simulink model "dnm_10_0"  (R2015a)
settings: Solver=ode3  StartTime=0.0  StopTime=100  FixedStep=0.001  RelTol=1e-3
libraries: slident x1, simulink x1
settings Model: Creator=Administrator  LastModifiedBy=Administrator
settings DataIOCC: LimitDataPoints=off

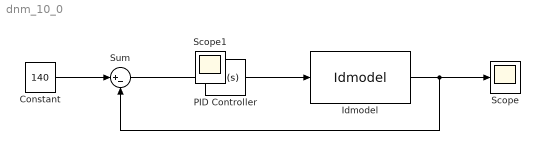
== system dnm_10_0 ==
  Constant : Constant  Value=140
  Idmodel : slident/Models/Idmodel  sys=P1Dc_10_0  IC=0  noi=off  seed=[]
  PID Controller : simulink/Continuous/PID Controller  Controller=PID  TimeDomain=Continuous-time  SampleTime=-1  IntegratorMethod=Forward Euler  FilterMethod=Forward Euler  Form=Parallel  UseFilter=on  ControllerParametersSource=internal  P=0.093556670716069  I=0.00376519243488328  D=0  N=100  InitialConditionSource=internal  InitialConditionForIntegrator=0  InitialConditionForFilter=0  ExternalReset=none  LimitOutput=off  UpperSaturationLimit=inf  LowerSaturationLimit=-inf  LinearizeAsGain=on  AntiWindupMode=none  Kb=1  TrackingMode=off  Kt=1  PParamMin=[]  PParamMax=[]  IParamMin=[]  IParamMax=[]  DParamMin=[]  DParamMax=[]  NParamMin=[]  NParamMax=[]  KbParamMin=[]  KbParamMax=[]  KtParamMin=[]  KtParamMax=[]  POutMin=[]  POutMax=[]  IOutMin=[]  IOutMax=[]  DOutMin=[]  DOutMax=[]  NOutMin=[]  NOutMax=[]  KbOutMin=[]  KbOutMax=[]  KtOutMin=[]  KtOutMax=[]  IntegratorOutMin=[]  IntegratorOutMax=[]  FilterOutMin=[]  FilterOutMax=[]  SumOutMin=[]  SumOutMax=[]  SumI1OutMin=[]  SumI1OutMax=[]  SumI2OutMin=[]  SumI2OutMax=[]  SumI3OutMin=[]  SumI3OutMax=[]  SumDOutMin=[]  SumDOutMax=[]  SaturationOutMin=[]  SaturationOutMax=[]  IntegratorContinuousStateAttributes=''  IntegratorStateMustResolveToSignalObject=off  IntegratorRTWStateStorageClass=Auto  FilterContinuousStateAttributes=''  FilterStateMustResolveToSignalObject=off  FilterRTWStateStorageClass=Auto  DifferentiatorICPrevScaledInput=0  DifferentiatorOutMin=[]  DifferentiatorOutMax=[]
  Scope : Scope
      settings: TimeRange=7.793113224224824e-05  YMin=7071565284414.506  YMax=10165830320824.72
  Sum : Sum  Inputs=|+-
  Scope1 : Scope
  wires:
  PID Controller/1 -> Idmodel/1
  Sum/1 -> PID Controller/1
  Idmodel/1 -> Scope/1, Sum/2
  Constant/1 -> Sum/1
